simulink model "Integ_Model_Hepta_Test"  (R2020b)
settings: configuration reference "VLS_Standard_Configuration" (kept outside this file)
settings Model: DataDictionary=Hepta_Integrated_SLDD.sldd  NumberOfSteps=5  Creator=ahashem  LastModifiedBy=yli69
settings ConfigSetRef: SourceName=VLS_Standard_Configuration

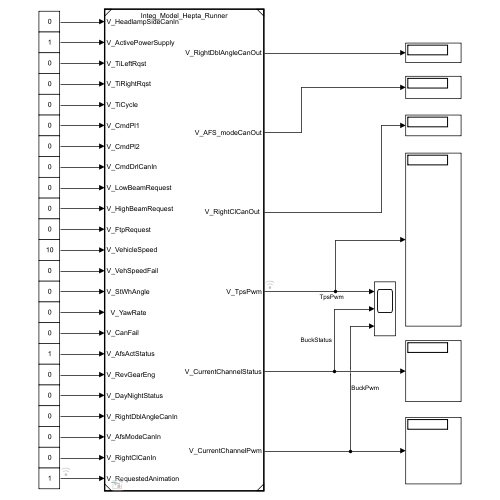
[thumbnail: Simulink's stored preview of the top-level diagram]
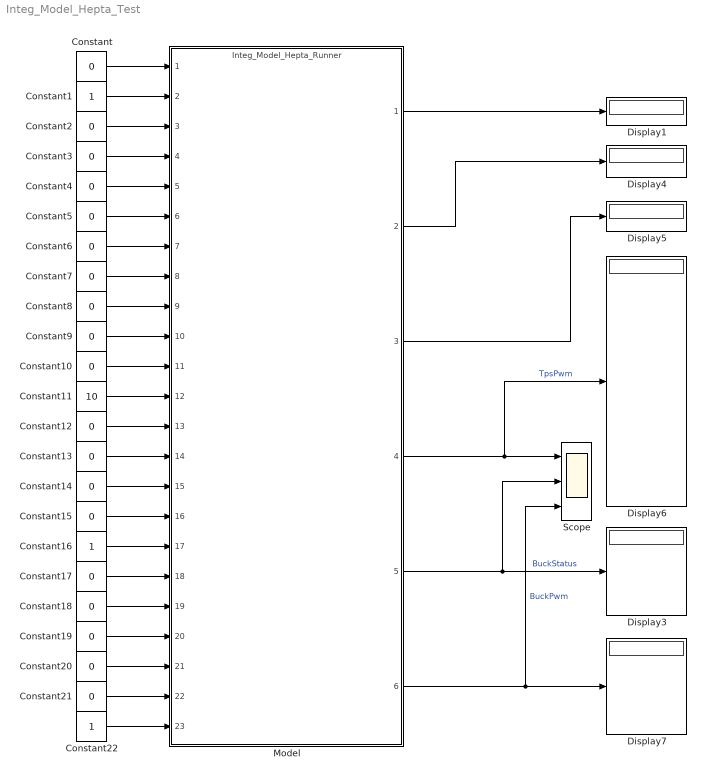
== system Integ_Model_Hepta_Test ==
  Constant{,2..10,12..15,17..21} (19 alike) : Constant  Value=0  OutDataTypeStr=Inherit: Inherit via back propagation
  Constant1 : Constant  OutDataTypeStr=Inherit: Inherit via back propagation
  Constant11 : Constant  Value=10  OutDataTypeStr=Inherit: Inherit via back propagation
  Constant16 : Constant  OutDataTypeStr=Inherit: Inherit via back propagation
  Constant22 : Constant  OutDataTypeStr=Inherit: Inherit via back propagation
  Display{1,3..7} (6 alike) : Display
  Model : ModelReference  ModelNameDialog=Integ_Model_Hepta_Runner.slx  SimulationMode=Normal  ModelReferenceVersion=4.4
  Scope : Scope  NumInputPorts=3
  wires:
  Model/4 -> Display6/1, Scope/1  "TpsPwm"
  Model/1 -> Display1/1
  Model/2 -> Display4/1
  Model/3 -> Display5/1
  Model/6 -> Scope/3, Display7/1  "BuckPwm"
  Model/5 -> Display3/1, Scope/2  "BuckStatus"
  Constant/1 -> Model/1
  Constant2/1 -> Model/3
  Constant1/1 -> Model/2
  Constant3/1 -> Model/4
  Constant4/1 -> Model/5
  Constant5/1 -> Model/6
  Constant6/1 -> Model/7
  Constant7/1 -> Model/8
  Constant8/1 -> Model/9
  Constant9/1 -> Model/10
  Constant10/1 -> Model/11
  Constant21/1 -> Model/22
  Constant15/1 -> Model/16
  Constant12/1 -> Model/13
  Constant14/1 -> Model/15
  Constant13/1 -> Model/14
  Constant19/1 -> Model/20
  Constant18/1 -> Model/19
  Constant16/1 -> Model/17
  Constant20/1 -> Model/21
  Constant11/1 -> Model/12
  Constant17/1 -> Model/18
  Constant22/1 -> Model/23
